simulink model "model_6ws6wd_2"  (R2023a)
settings: Solver=VariableStepAuto  StartTime=0.0  StopTime=10.0  RelTol=1e-3
settings Model: Creator=NGOC MAI  LastModifiedBy=NGOC MAI

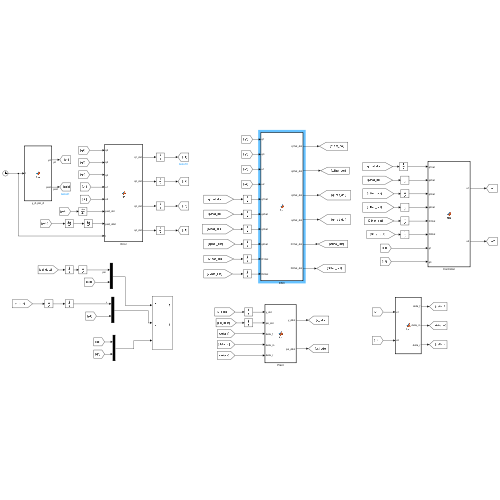
[thumbnail: Simulink's stored preview of the top-level diagram]
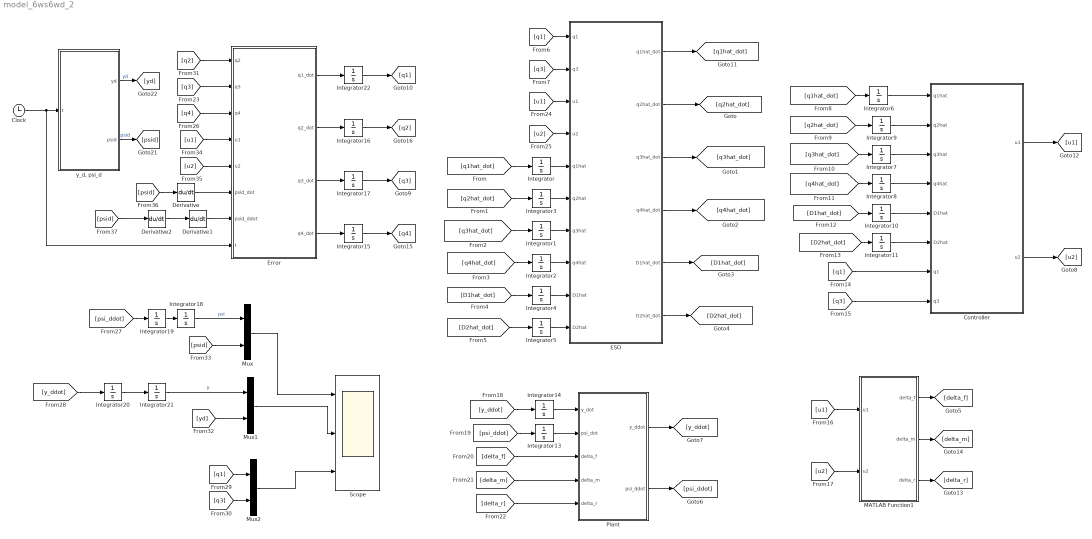
== system model_6ws6wd_2 ==
  Clock : Clock
  Controller : MATLAB Function  TreatAsAtomicUnit=on
  Derivative : Derivative
  Derivative1 : Derivative
  Derivative2 : Derivative
  ESO : MATLAB Function  TreatAsAtomicUnit=on
  Error : MATLAB Function  TreatAsAtomicUnit=on
  Integrator{,1..11,13..22} (22 alike) : Integrator
  MATLAB Function1 : MATLAB Function  TreatAsAtomicUnit=on
  Mux : Mux  Inputs=2
  Mux1 : Mux  Inputs=2
  Mux2 : Mux  Inputs=2
  Plant : MATLAB Function  TreatAsAtomicUnit=on
  Scope : Scope  NumInputPorts=3
  "y_d, psi_d" : MATLAB Function  TreatAsAtomicUnit=on
  wires:
  Clock/1 -> Error/8(t), "y_d, psi_d"/1(t)
  ESO/5(D1hat_dot) -> [D1hat_dot]
  ESO/6(D2hat_dot) -> [D2hat_dot]
  ESO/4(q4hat_dot) -> [q4hat_dot]
  ESO/3(q3hat_dot) -> [q3hat_dot]
  ESO/2(q2hat_dot) -> [q2hat_dot]
  ESO/1(q1hat_dot) -> [q1hat_dot]
  Integrator/1 -> ESO/5(q1hat)
  Integrator3/1 -> ESO/6(q2hat)
  Integrator1/1 -> ESO/7(q3hat)
  Integrator2/1 -> ESO/8(q4hat)
  [q1hat_dot] -> Integrator/1
  [q3hat_dot] -> Integrator1/1
  [q2hat_dot] -> Integrator3/1
  [q4hat_dot] -> Integrator2/1
  Integrator5/1 -> ESO/10(D2hat)
  Integrator4/1 -> ESO/9(D1hat)
  [D1hat_dot] -> Integrator4/1
  [D2hat_dot] -> Integrator5/1
  [q1] -> ESO/1(q1)
  [q3] -> ESO/2(q3)
  [q3hat_dot] -> Integrator7/1
  Integrator11/1 -> Controller/6(D2hat)
  Integrator6/1 -> Controller/1(q1hat)
  [D1hat_dot] -> Integrator10/1
  [q4hat_dot] -> Integrator8/1
  Integrator10/1 -> Controller/5(D1hat)
  Integrator7/1 -> Controller/3(q3hat)
  Integrator8/1 -> Controller/4(q4hat)
  [q1hat_dot] -> Integrator6/1
  [D2hat_dot] -> Integrator11/1
  [q2hat_dot] -> Integrator9/1
  Integrator9/1 -> Controller/2(q2hat)
  [q1] -> Controller/7(q1)
  [q3] -> Controller/8(q3)
  Controller/1(u1) -> [u1]
  Controller/2(u2) -> [u2]
  [u1] -> MATLAB Function1/1(u1)
  [u2] -> MATLAB Function1/2(u2)
  Integrator14/1 -> Plant/1(y_dot)
  [y_ddot] -> Integrator14/1
  [psi_ddot] -> Integrator13/1
  Integrator13/1 -> Plant/2(psi_dot)
  Plant/1(y_ddot) -> [y_ddot]
  Plant/2(psi_ddot) -> [psi_ddot]
  MATLAB Function1/1(delta_f) -> [delta_f]
  MATLAB Function1/2(delta_m) -> [delta_m]
  MATLAB Function1/3(delta_r) -> [delta_r]
  [delta_f] -> Plant/3(delta_f)
  [delta_m] -> Plant/4(delta_m)
  [delta_r] -> Plant/5(delta_r)
  [u1] -> ESO/3(u1)
  [u2] -> ESO/4(u2)
  [psi_ddot] -> Integrator19/1
  Integrator19/1 -> Integrator18/1
  Integrator20/1 -> Integrator21/1
  [y_ddot] -> Integrator20/1
  Integrator18/1 -> Mux/1  "psi"
  Integrator21/1 -> Mux1/1  "y"
  Mux/1 -> Scope/1
  Mux1/1 -> Scope/2
  [q1] -> Mux2/1
  [q3] -> Mux2/2
  Mux2/1 -> Scope/3
  Error/1(q1_dot) -> Integrator22/1
  Integrator22/1 -> [q1]
  Error/3(q3_dot) -> Integrator17/1
  Integrator17/1 -> [q3]
  [q3] -> Error/2(q3)
  Error/4(q4_dot) -> Integrator15/1
  Integrator15/1 -> [q4]
  [q4] -> Error/3(q4)
  Error/2(q2_dot) -> Integrator16/1
  Integrator16/1 -> [q2]
  [q2] -> Error/1(q2)
  "y_d, psi_d"/1(yd) -> [yd]  "yd"
  [yd] -> Mux1/2
  "y_d, psi_d"/2(psid) -> [psid]  "psid"
  [psid] -> Mux/2
  [u1] -> Error/4(u1)
  [u2] -> Error/5(u2)
  [psid] -> Derivative/1
  Derivative/1 -> Error/6(psid_dot)
  [psid] -> Derivative2/1
  Derivative2/1 -> Derivative1/1
  Derivative1/1 -> Error/7(psid_ddot)

== matlab function model_6ws6wd_2/Error ==
  data: q2 input; q1_dot output; q3 input; q4 input; u1 input; q2_dot output; u2 input; psid_dot input; psid_ddot input; t input; q3_dot output; q4_dot output
function [q1_dot,q2_dot,q3_dot,q4_dot]= fcn(q2,q3,q4,u1,u2,psid_dot,psid_ddot,t)
m=1350; %kg
J=1350; %kgm^2
cf=55000; %N/rad
cm=100000; %N/rad
cr=120000; %N/rad
lf=2.5; %m
lm=0.5; %m
lr=3; %m
vx=20; %m/s

m1=2*(-cf-cr-cm)/(m*vx);
m2=2*(cf+cr+cm)/m;
m3=2*(lf*cf+lr*cr+lm*cm)/(m*vx);
m4=m3;
n1=2*(-lf*cf+lr*cr-lm*cm)/(J*vx);
n2=2*(lf*cf-lr*cr+lm*cm)/J;
n3=2*((lf^2)*cf+(lm^2)*cm-(lr^2)*cr)/(J*vx);
n4=n3;
D1=9.8*cos(10)+m4*psid_dot+3*sin(t)+cos(t/2);
D2=-psid_ddot+n4*psid_dot+2.5*sin(t)-cos(t);
q1_dot=q2;
q2_dot=m1*q2+m2*q3+m3*q4+u1+D1;
q3_dot=q4;
q4_dot=n1*q2+n2*q3+n3*q4+u2+D2;
end

== matlab function model_6ws6wd_2/Plant ==
  data: y_dot input; y_ddot output; psi_dot input; delta_f input; delta_m input; psi_ddot output; delta_r input
function [y_ddot,psi_ddot] = fcn(y_dot,psi_dot,delta_f,delta_m,delta_r)
m=1350; %kg
J=1350; %kgm^2
cf=55000; %N/rad
cm=100000; %N/rad
cr=120000; %N/rad
lf=2.5; %m
lm=0.5; %m
lr=3; %m
vx=20; %m/s
k1=(-2*cf-2*cr-2*cm)/(m*vx);
k2=2*(lf*cf+lr*cr+lm*cm)/(m*vx)-vx;
k3=2*(-lf*cf+lr*cr-lm*cm)/(J*vx);
k4=2*((lf^2)*cf-(lr^2)*cr+(lm^2)*cm)/(J*vx);
d1=9.8*cos(10);
u1=2*(cf*delta_f+cm*delta_m+cr*delta_r)/m;
u2=2*(lf*cf*delta_f+lm*cm*delta_m-lr*cr*delta_r)/J;
y_ddot=k1*y_dot+k2*psi_dot+u1+d1;
psi_ddot=k3*y_dot+k4*psi_dot+u2;
end

== matlab function model_6ws6wd_2/ESO ==
  data: q1 input; q1hat_dot output; q3 input; u1 input; u2 input; q1hat input; q2hat input; q3hat input; q4hat input; D1hat input; D2hat input; q2hat_dot output; q3hat_dot output; q4hat_dot output; D1hat_dot output; D2hat_dot output
function [q1hat_dot,q2hat_dot,q3hat_dot,q4hat_dot,D1hat_dot,D2hat_dot]= fcn(q1,q3,u1,u2,q1hat,q2hat,q3hat,q4hat,D1hat,D2hat)
m=1350; %kg
J=1350; %kgm^2
cf=55000; %N/rad
cm=100000; %N/rad
cr=120000; %N/rad
lf=2.5; %m
lm=0.5; %m
lr=3; %m
vx=20; %m/s

m1=2*(-cf-cr-cm)/(m*vx);
m2=2*(cf+cr+cm)/m;
m3=2*(lf*cf+lr*cr+lm*cm)/(m*vx);
n1=2*(-lf*cf+lr*cr-lm*cm)/(J*vx);
n2=2*(lf*cf-lr*cr+lm*cm)/J;
n3=2*((lf^2)*cf+(lm^2)*cm-(lr^2)*cr)/(J*vx);
a1=6;
a2=11;
a3=6;
epsi1=0.027;
epsi2=0.01;

q1hat_dot=q2hat+a1*(q1-q1hat)/epsi1;
q2hat_dot=D1hat+m1*q2hat+m2*q3hat+m3*q4hat+u1+a2*(q1-q1hat)/(epsi1^2);
D1hat_dot=a3*(q1-q1hat)/(epsi1^3);
q3hat_dot=q4hat+a1*(q3-q3hat)/epsi2;
q4hat_dot=D2hat+n1*q2hat+n2*q3hat+n3*q4hat+u2+a2*(q3-q3hat)/(epsi2^2);
D2hat_dot=a3*(q3-q3hat)/epsi2^3;
end

== matlab function model_6ws6wd_2/y_d, psi_d ==
  data: t input; yd output; psid output
function [yd,psid]= fcn(t)
%yd=10*(tanh(3*t-35)-tanh(3*t-6));
%psid=(sech(3*t-60))^2-(sech(3*t-35)^2);
yd = 1.5*(tanh(t-6) - tanh(t-14));
psid = 1.5*(-(sech(t-14))^2 + (sech(t-6))^2)/20;
end

== matlab function model_6ws6wd_2/Controller ==
  data: u1 output; u2 output; q1hat input; q2hat input; q3hat input; q4hat input; D1hat input; D2hat input; q1 input; q3 input
function [u1, u2]= fcn(q1hat,q2hat,q3hat,q4hat,D1hat,D2hat,q1,q3)
%a1=6;
a2=11;
%a3=6;
epsi1=0.027;
epsi2=0.01;
p1=12;
p2=25;
c1=3;
c2=0.5;
c3=2;
c4=4;

m=1350; %kg
J=1350; %kgm^2
cf=55000; %N/rad
cm=100000; %N/rad
cr=120000; %N/rad
lf=2.5; %m
lm=0.5; %m
lr=3; %m
vx=20; %m/s

m1=2*(-cf-cr-cm)/(m*vx);
m2=2*(cf+cr+cm)/m;
m3=2*(lf*cf+lr*cr+lm*cm)/(m*vx);
%D1=9.8*cos(10)+m4*psid_dot+3*sin(t)+cos(t/2);
n1=2*(-lf*cf+lr*cr-lm*cm)/(J*vx);
n2=2*(lf*cf-lr*cr+lm*cm)/J;
n3=2*((lf^2)*cf+(lm^2)*cm-(lr^2)*cr)/(J*vx);
s1=p1*q1hat+q2hat;
s2=p2*q3hat+q4hat;

u1=-c1*s1-c2*sat(s1)-p1*q2hat-D1hat-m1*q2hat-m2*q3hat-m3*q4hat-a2*(q1-q1hat)/epsi1^2;
u2=-c3*s2-c4*sat(s2)-p2*q4hat-D2hat-n1*q2hat-n2*q3hat-n3*q4hat-a2*(q3-q3hat)/epsi2^2;
end

== matlab function model_6ws6wd_2/MATLAB Function1 ==
  data: u1 input; delta_f output; u2 input; delta_m output; delta_r output
function [delta_f,delta_m,delta_r] = fcn(u1,u2)
m=1350; %kg
J=1350; %kgm^2
cf=55000; %N/rad
cm=100000; %N/rad
cr=120000; %N/rad
lf=2.5; %m
lm=0.5; %m
lr=3; %m
%vx=20; %m/s
A=[cf cm cr;cf*lf cm*lm -cr*lr;1/2 -1 1/2];
B=[u1*m/2;u2*J/2;0];
C=A^(-1)*B;
delta_f=C(1,1);
delta_m=C(2,1);
delta_r=C(3,1);
end
